simulink model "PubIfDecisionTOS_MDL"  (R2020b)
settings: configuration reference "DspaceConfig" (kept outside this file)
PostLoadFcn:
  | if any(exist('dsrtsu_mdlpostloadfcn', 'file') ~= 0), dsrtsu_mdlpostloadfcn('Execute', bdroot); end
InitFcn:
  | , if any(exist('dsmpb_private', 'file') ~= 0), dsmpb_private('dsmpb_mdlclblib', 'Init', bdroot); end,
undefined symbols (not defined in the file or in its folder): C_TOS_ACCEgoRAxletoFbumplength_m, C_TOS_ACCTargetFront_Flag, C_TOS_AEBJAPedObjDxThre_Val, C_TOS_AEBJAPedObjDyThre_Val, C_TOS_AEBJATargetSize_Val, C_TOS_AEBJAVehObjDxThre_Val, C_TOS_AEBJAVehObjDyThre_Val, C_TOS_AEBJuncPedTargetSize_Val, C_TOS_AEBLatObjDxThre_Val, C_TOS_AEBLatPedDyThre_Val, C_TOS_AEBLatTargetSize_Val, C_TOS_AEBLongTargetInEgoFront_Flag, C_TOS_axAbsGround_Parameter, C_TOS_CameraConfirmedFlag, C_TOS_CNsubjWidth, C_TOS_CurrentLaneCoreMinWidth_Val, C_TOS_CutInProb_Val_Zero, C_TOS_CutOutProb_Val_Zero, C_TOS_D2R_Val, C_TOS_DefaultValueObjectToCenterLine_dy, C_TOS_EgoCarWidth_Val, C_TOS_EgoDxRefPoint_m, C_TOS_EgoRAxletoFbumplength_m, C_TOS_HalfWidthVehicle_Con, C_TOS_HWA_CurrentLaneFlag, C_TOS_HWA_LeftLaneFlag, C_TOS_HWA_MovingDir_Vaild, C_TOS_HWA_MovState_Vaild, C_TOS_HWA_RightLaneFlag, C_TOS_LaneLineCourseErrorFront, C_TOS_LaneLineCourseErrorRear, C_TOS_MotorbikeDefaultWidth_m, C_TOS_NumberOfEffectiveTargets, C_TOS_Obj_Age_Val, C_TOS_Objdx_Constraint_Val, C_TOS_ObjectDefaultWidth_m, C_TOS_ObjInCurrentLane_Val, C_TOS_ObjInCurrentLaneValid, C_TOS_ObjInLeftLaneValid, C_TOS_ObjInRightLaneValid, C_TOS_ObjNotInCurrentLane_Val, C_TOS_ObjNotREElementType, C_TOS_ObjPredictDis_dy_ConstantVal_Zeros, C_TOS_ObjToCenterLine_ConstantVal_Zeros, C_TOS_OFMObjIDInvilad_Val, C_TOS_PIL_LatDisCons_Val_zero, C_TOS_PIL_ObjectCutInFlag_b, C_TOS_PIL_ObjectCutOutFlag_b, C_TOS_PIL_ObjLaneProb_al_Val, C_TOS_PP_ObjFusType_FC_Confirm_b, C_TOS_PP_ObjFusType_FC_FR_Confirm_b, C_TOS_PP_ObjFusType_FR_Confirm_b, C_TOS_RE_80BoolDefault_Val, C_TOS_RE_80Single181Default_Val, C_TOS_RE_80Single255Default_Val, C_TOS_RE_80Uint8Default_Val, C_TOS_RE_D2R, C_TOS_RE_D_180_Val, C_TOS_RE_InvalidObjectID_Val, C_TOS_RE_InvalidTargetChainDir_Val ... (+142)
libraries: simulink x1650, TOS_LIB x361, canfdmsglib x14
(part 69 of 69)

== stateflow chart PubIfDecisionTOS_MDL/TOS_20201112/TOS_2012080320/TOS/LC_LCKie_ELK/HWA_TargetInfor/TOS_HWA_TargetInfor ==
  (default) -> (junction 140) : {i = uint8(1);}
  (junction 140) -> (junction 145) [order 1] : [i <= P_TOS_LCTargetNum_Val]
  (junction 147) -> (junction 140) : {i=i+uint8(1);}
  (junction 140) -> (junction 143) [order 2]
  (junction 145) -> (junction 147) : {
      | TOS_LCTargetInfor.Object_Fus_Type(i) = uint8(0);
      | TOS_LCTargetInfor.Object_ID(i) = uint8(0);
      | TOS_LCTargetInfor.Object_Type(i) = uint8(0);
      | TOS_LCTargetInfor.Object_Length(i) = single(0);
      | TOS_LCTargetInfor.Object_Width(i) = single(0);
      | TOS_LCTargetInfor.Object_Hight(i) =single(0);
      | TOS_LCTargetInfor.Object_HeadingAngle(i) =single(0);
      | TOS_LCTargetInfor.Object_YawAngle(i) = single(0);
      | TOS_LCTargetInfor.Object_MovingState(i) = uint8(0);
      | TOS_LCTargetInfor.Object_Orientation(i) = uint8(0);
      | TOS_LCTargetInfor.Object_DX(i) = single(0);
      | TOS_LCTargetInfor.Object_DY(i) = single(0);
      | TOS_LCTargetInfor.Object_VX(i) = single(0);
      | TOS_LCTargetInfor.Object_VY(i) = single(0);
      | TOS_LCTargetInfor.Object_Std_AX(i) = single(0);
      | TOS_LCTargetInfor.Object_Std_AY(i) = single(0);
      | TOS_LCTargetInfor.Object_Std_DX(i) = single(0);
      | TOS_LCTargetInfor.Object_Std_DY(i) = single(0);
      | TOS_LCTargetInfor.Object_Std_VX(i) = single(0);
      | TOS_LCTargetInfor.Object_Std_VY(i) = single(0);
      | TOS_LCTargetInfor.Object_AX(i) = single(0);
      | TOS_LCTargetInfor.Object_AY(i) = single(0);
      | TOS_LCTargetInfor.Object_Std_Length(i) = single(0);
      | TOS_LCTargetInfor.Object_Std_Width(i) = single(0);
      | TOS_LCTargetInfor.Object_Std_HeadingAngle(i) = single(0);
      | TOS_LCTargetInfor.Object_Type_Prob(i) = single(0);
      | TOS_LCTargetInfor.Object_ExistProb(i) = single(0);
      | TOS_LCTargetInfor.Object_ObstacleProb(i) = single(0);
      | TOS_LCTargetInfor.Object_Age(i) = uint16(0);
      | TOS_LCTargetInfor.CurrentLane_Prob(i) = single(0);
      | TOS_LCTargetInfor.LeftLane_Prob(i) = single(0);
      | TOS_LCTargetInfor.RightLane_Prob(i) = single(0);
      | TOS_LCTargetInfor.ObjectIn_Lane(i) = uint8(0);
      | }
  (junction 143) -> (junction 56)
  (junction 56) -> (junction 121) : {i=uint8(1);
      | TargetIndex = uint8(0);}
  (junction 121) -> (junction 122) [order 1] : [i <= P_TOS_LCTargetNum_Val]
  (junction 124) -> (junction 121) : {i=i+uint8(1);}
  (junction 121) -> (junction 127) [order 2]
  (junction 122) -> (junction 158)
  (junction 158) -> (junction 160) [order 1] : [TOS_HWA_TargetIndexVector(i)~=uint8(0)]
  (junction 158) -> (junction 163) [order 2]
  (junction 160) -> (junction 162) : {TargetIndex=TOS_HWA_TargetIndexVector(i);
      | TOS_LCTargetInfor.Object_Fus_Type(i) = OFM_SignalVerification.Object_Fus_Type(TargetIndex);
      | TOS_LCTargetInfor.Object_ID(i) = OFM_SignalVerification.Object_ID(TargetIndex);
      | TOS_LCTargetInfor.Object_Type(i) = OFM_SignalVerification.Object_Type(TargetIndex);
      | TOS_LCTargetInfor.Object_Length(i) = OFM_SignalVerification.Object_Length(TargetIndex);
      | TOS_LCTargetInfor.Object_Width(i) = OFM_SignalVerification.Object_Width(TargetIndex);
      | TOS_LCTargetInfor.Object_Hight(i) = OFM_SignalVerification.Object_Hight(TargetIndex);
      | TOS_LCTargetInfor.Object_HeadingAngle(i) = OFM_SignalVerification.Object_HeadingAngle(TargetIndex);
      | TOS_LCTargetInfor.Object_YawAngle(i) = OFM_SignalVerification.Object_YawAngle(TargetIndex);
      | TOS_LCTargetInfor.Object_MovingState(i) = TOS_AddAttributes.PP_MovingStateSignalProcessing(TargetIndex);
      | TOS_LCTargetInfor.Object_Orientation(i) = TOS_AddAttributes.PP_ObjMovingDirSignalProcessing(TargetIndex);
      | TOS_LCTargetInfor.Object_DX(i) = OFM_SignalVerification.Object_DX(TargetIndex);
      | TOS_LCTargetInfor.Object_DY(i) = OFM_SignalVerification.Object_DY(TargetIndex);
      | TOS_LCTargetInfor.Object_VX(i) = OFM_SignalVerification.Object_VX(TargetIndex);
      | TOS_LCTargetInfor.Object_VY(i) = OFM_SignalVerification.Object_VY(TargetIndex);
      | TOS_LCTargetInfor.Object_Std_AX(i) = OFM_SignalVerification.Object_Std_AX(TargetIndex);
      | TOS_LCTargetInfor.Object_Std_AY(i) = OFM_SignalVerification.Object_Std_AY(TargetIndex);
      | TOS_LCTargetInfor.Object_Std_DX(i) = OFM_SignalVerification.Object_Std_DX(TargetIndex);
      | TOS_LCTargetInfor.Object_Std_DY(i) = OFM_SignalVerification.Object_Std_DY(TargetIndex);
      | TOS_LCTargetInfor.Object_Std_VX(i) = OFM_SignalVerification.Object_Std_VX(TargetIndex);
      | TOS_LCTargetInfor.Object_Std_VY(i) = OFM_SignalVerification.Object_Std_VY(TargetIndex);
      | TOS_LCTargetInfor.Object_AX(i) = OFM_SignalVerification.Object_AX(TargetIndex);
      | TOS_LCTargetInfor.Object_AY(i) = OFM_SignalVerification.Object_AY(TargetIndex);
      | TOS_LCTargetInfor.Object_Std_Length(i) = OFM_SignalVerification.Object_Std_Length(TargetIndex);
      | TOS_LCTargetInfor.Object_Std_Width(i) = OFM_SignalVerification.Object_Std_Width(TargetIndex);
      | TOS_LCTargetInfor.Object_Std_HeadingAngle(i) = OFM_SignalVerification.Object_Std_HeadingAngle(TargetIndex);
      | TOS_LCTargetInfor.Object_Type_Prob(i) = OFM_SignalVerification.Object_Type_Prob(TargetIndex);
      | TOS_LCTargetInfor.Object_ExistProb(i) = OFM_SignalVerification.Object_ExistProb(TargetIndex);
      | TOS_LCTargetInfor.Object_ObstacleProb(i) = OFM_SignalVerification.Object_ObstacleProb(TargetIndex);
      | TOS_LCTargetInfor.Object_Age(i) = OFM_SignalVerification.Object_Age(TargetIndex);
      | TOS_LCTargetInfor.CurrentLane_Prob(i) = TOS_ProbInLaneCalculat.PIL_CurrentLaneProb(TargetIndex);
      | TOS_LCTargetInfor.LeftLane_Prob(i) = TOS_ProbInLaneCalculat.PIL_LeftLaneProb(TargetIndex);
      | TOS_LCTargetInfor.RightLane_Prob(i) = TOS_ProbInLaneCalculat.PIL_RightLaneProb(TargetIndex);
      | TOS_LCTargetInfor.ObjectIn_Lane(i) =  ObjectIn_Lane_b(i);
      | }
  (junction 162) -> (junction 163)
  (junction 163) -> (junction 124)
  (junction 127) -> (junction 129)
  data: OFM_SignalVerification input Bus: OFM_OBJ_BUS; TOS_AddAttributes input Bus: TOS_AddAttributes_BUS; TOS_ProbInLaneCalculat input Bus: PIL_ProbInLaneCalculat_BUS; ObjectIn_Lane_b input uint8; TOS_HWA_TargetIndexVector input size=11; TOS_LCTargetInfor output Bus: TOS_LC_BUS size=1 =0; P_TOS_LCTargetNum_Val parameter uint8; TargetIndex local uint8 size=1; i local uint8 size=1

== stateflow chart PubIfDecisionTOS_MDL/TOS_20201112/TOS_2012080320/TOS/LC_LCKie_ELK/LCKie_TargetInfor/TOS_LCKieTargetInfor ==
  (default) -> (junction 161) : {i = uint8(1);}
  (junction 161) -> (junction 166) [order 1] : [i <= P_TOS_LCKieTargetNum_Val]
  (junction 169) -> (junction 161) : {i=i+uint8(1);}
  (junction 161) -> (junction 157) [order 2]
  (junction 166) -> (junction 169) : {
      | TOS_LCKieTargetInfor.Object_Fus_Type(i) = uint8(0);
      | TOS_LCKieTargetInfor.Object_ID(i) = uint8(0);
      | TOS_LCKieTargetInfor.Object_Type(i) = uint8(0);
      | TOS_LCKieTargetInfor.Object_Length(i) = single(0);
      | TOS_LCKieTargetInfor.Object_Width(i) = single(0);
      | TOS_LCKieTargetInfor.Object_Hight(i) =single(0);
      | TOS_LCKieTargetInfor.Object_HeadingAngle(i) =single(0);
      | TOS_LCKieTargetInfor.Object_YawAngle(i) = single(0);
      | TOS_LCKieTargetInfor.Object_MovingState(i) = uint8(0);
      | TOS_LCKieTargetInfor.Object_Orientation(i) = uint8(0);
      | TOS_LCKieTargetInfor.Object_DX(i) = single(0);
      | TOS_LCKieTargetInfor.Object_DY(i) = single(0);
      | TOS_LCKieTargetInfor.Object_VX(i) = single(0);
      | TOS_LCKieTargetInfor.Object_VY(i) = single(0);
      | TOS_LCKieTargetInfor.Object_Std_AX(i) = single(0);
      | TOS_LCKieTargetInfor.Object_Std_AY(i) = single(0);
      | TOS_LCKieTargetInfor.Object_Std_DX(i) = single(0);
      | TOS_LCKieTargetInfor.Object_Std_DY(i) = single(0);
      | TOS_LCKieTargetInfor.Object_Std_VX(i) = single(0);
      | TOS_LCKieTargetInfor.Object_Std_VY(i) = single(0);
      | TOS_LCKieTargetInfor.Object_AX(i) = single(0);
      | TOS_LCKieTargetInfor.Object_AY(i) = single(0);
      | TOS_LCKieTargetInfor.Object_Std_Length(i) = single(0);
      | TOS_LCKieTargetInfor.Object_Std_Width(i) = single(0);
      | TOS_LCKieTargetInfor.Object_Std_HeadingAngle(i) = single(0);
      | TOS_LCKieTargetInfor.Object_Type_Prob(i) = single(0);
      | TOS_LCKieTargetInfor.Object_ExistProb(i) = single(0);
      | TOS_LCKieTargetInfor.Object_ObstacleProb(i) = single(0);
      | TOS_LCKieTargetInfor.Object_Age(i) = uint16(0);
      | TOS_LCKieTargetInfor.cutIn(i) = uint8(0);
      | TOS_LCKieTargetInfor.CurrentLane_Prob(i) = single(0);
      | TOS_LCKieTargetInfor.LeftLane_Prob(i) = single(0);
      | TOS_LCKieTargetInfor.RightLane_Prob(i) = single(0);
      | TOS_LCKieTargetInfor.ObjectIn_Lane(i) = uint8(0);
      | }
  (junction 157) -> (junction 178)
  (junction 178) -> (junction 184) : {i=uint8(1);
      | TargetIndex = uint8(0);}
  (junction 184) -> (junction 155) [order 1] : [i <= P_TOS_LCKieTargetNum_Val]
  (junction 180) -> (junction 184) : {i=i+uint8(1);}
  (junction 184) -> (junction 181) [order 2]
  (junction 155) -> (junction 174)
  (junction 174) -> (junction 159) [order 1] : [TOS_HWA_TargetIndexVector(i)~=uint8(0)]
  (junction 174) -> (junction 170) [order 2]
  (junction 159) -> (junction 173) : {TargetIndex=TOS_HWA_TargetIndexVector(i);
      | TOS_LCKieTargetInfor.Object_Fus_Type(i) = OFM_SignalVerification.Object_Fus_Type(TargetIndex);
      | TOS_LCKieTargetInfor.Object_ID(i) = OFM_SignalVerification.Object_ID(TargetIndex);
      | TOS_LCKieTargetInfor.Object_Type(i) = OFM_SignalVerification.Object_Type(TargetIndex);
      | TOS_LCKieTargetInfor.Object_Length(i) = OFM_SignalVerification.Object_Length(TargetIndex);
      | TOS_LCKieTargetInfor.Object_Width(i) = OFM_SignalVerification.Object_Width(TargetIndex);
      | TOS_LCKieTargetInfor.Object_Hight(i) = OFM_SignalVerification.Object_Hight(TargetIndex);
      | TOS_LCKieTargetInfor.Object_HeadingAngle(i) = OFM_SignalVerification.Object_HeadingAngle(TargetIndex);
      | TOS_LCKieTargetInfor.Object_YawAngle(i) = OFM_SignalVerification.Object_YawAngle(TargetIndex);
      | TOS_LCKieTargetInfor.Object_MovingState(i) = TOS_AddAttributes.PP_MovingStateSignalProcessing(TargetIndex);
      | TOS_LCKieTargetInfor.Object_Orientation(i) = TOS_AddAttributes.PP_ObjMovingDirSignalProcessing(TargetIndex);
      | TOS_LCKieTargetInfor.Object_DX(i) = OFM_SignalVerification.Object_DX(TargetIndex);
      | TOS_LCKieTargetInfor.Object_DY(i) = OFM_SignalVerification.Object_DY(TargetIndex);
      | TOS_LCKieTargetInfor.Object_VX(i) = OFM_SignalVerification.Object_VX(TargetIndex);
      | TOS_LCKieTargetInfor.Object_VY(i) = OFM_SignalVerification.Object_VY(TargetIndex);
      | TOS_LCKieTargetInfor.Object_Std_AX(i) = OFM_SignalVerification.Object_Std_AX(TargetIndex);
      | TOS_LCKieTargetInfor.Object_Std_AY(i) = OFM_SignalVerification.Object_Std_AY(TargetIndex);
      | TOS_LCKieTargetInfor.Object_Std_DX(i) = OFM_SignalVerification.Object_Std_DX(TargetIndex);
      | TOS_LCKieTargetInfor.Object_Std_DY(i) = OFM_SignalVerification.Object_Std_DY(TargetIndex);
      | TOS_LCKieTargetInfor.Object_Std_VX(i) = OFM_SignalVerification.Object_Std_VX(TargetIndex);
      | TOS_LCKieTargetInfor.Object_Std_VY(i) = OFM_SignalVerification.Object_Std_VY(TargetIndex);
      | TOS_LCKieTargetInfor.Object_AX(i) = OFM_SignalVerification.Object_AX(TargetIndex);
      | TOS_LCKieTargetInfor.Object_AY(i) = OFM_SignalVerification.Object_AY(TargetIndex);
      | TOS_LCKieTargetInfor.Object_Std_Length(i) = OFM_SignalVerification.Object_Std_Length(TargetIndex);
      | TOS_LCKieTargetInfor.Object_Std_Width(i) = OFM_SignalVerification.Object_Std_Width(TargetIndex);
      | TOS_LCKieTargetInfor.Object_Std_HeadingAngle(i) = OFM_SignalVerification.Object_Std_HeadingAngle(TargetIndex);
      | TOS_LCKieTargetInfor.Object_Type_Prob(i) = OFM_SignalVerification.Object_Type_Prob(TargetIndex);
      | TOS_LCKieTargetInfor.Object_ExistProb(i) = OFM_SignalVerification.Object_ExistProb(TargetIndex);
      | TOS_LCKieTargetInfor.Object_ObstacleProb(i) = OFM_SignalVerification.Object_ObstacleProb(TargetIndex);
      | TOS_LCKieTargetInfor.Object_Age(i) = OFM_SignalVerification.Object_Age(TargetIndex);
      | TOS_LCKieTargetInfor.cutIn(i) =TOS_ProbInLaneCalculat.PIL_CutinFlag(TargetIndex) ;
      | TOS_LCKieTargetInfor.CurrentLane_Prob(i) = TOS_ProbInLaneCalculat.PIL_CurrentLaneProb(TargetIndex);
      | TOS_LCKieTargetInfor.LeftLane_Prob(i) = TOS_ProbInLaneCalculat.PIL_LeftLaneProb(TargetIndex);
      | TOS_LCKieTargetInfor.RightLane_Prob(i) = TOS_ProbInLaneCalculat.PIL_RightLaneProb(TargetIndex);
      | TOS_LCKieTargetInfor.ObjectIn_Lane(i) = ObjectIn_Lane_b(i);
      | }
  (junction 173) -> (junction 170)
  (junction 170) -> (junction 180)
  (junction 181) -> (junction 158)
  data: OFM_SignalVerification input Bus: OFM_OBJ_BUS; TOS_AddAttributes input Bus: TOS_AddAttributes_BUS; TOS_ProbInLaneCalculat input Bus: PIL_ProbInLaneCalculat_BUS; ObjectIn_Lane_b input uint8; TOS_HWA_TargetIndexVector input size=11; TOS_LCKieTargetInfor output Bus: TOS_LCKIE_BUS size=1 =0; P_TOS_LCKieTargetNum_Val parameter uint8; TargetIndex local uint8 size=1; i local uint8 size=1

== matlab function PubIfDecisionTOS_MDL/TOS_20201112/TOS_2012080320/TOS/LC_LCKie_ELK/TOS_HWA/CurrentLane/HWA_CurrentLane ==
  data: F_Dx2edNearestObjIndex output; Object_Dx input; Object_ID input; F_Dx1stNearestObjIndex output; R_Dx1stNearestObjIndex output; R_Dx2edNearestObjIndex output; F_Dx1stNearestObjID output; F_Dx2edNearestObjID output; ConditionJudge input; TOS_HWA_CLF_TargetPre_Filt_Flag input; Object_Num input; R_Dx1stNearestObjID output; R_Dx2edNearestObjID output

%%%%ObjDisIndex按Dx从小到大的总排序
%%%%%%%%ObjectID按Dx从小到大的总排序
function [F_Dx2edNearestObjIndex,F_Dx1stNearestObjIndex,R_Dx1stNearestObjIndex,R_Dx2edNearestObjIndex,F_Dx1stNearestObjID,F_Dx2edNearestObjID,R_Dx1stNearestObjID,R_Dx2edNearestObjID]   = MinMax(Object_Dx,Object_ID,ConditionJudge,TOS_HWA_CLF_TargetPre_Filt_Flag, Object_Num)
Dx_Front = Object_Dx;
Dx_Rear = Object_Dx;
ID = Object_ID;
for i=int32(1):int32(Object_Num)
    
    if (ID(i) == uint8(0))||(ConditionJudge(i) == false)||(Dx_Front(i) < single(0)) ||(TOS_HWA_CLF_TargetPre_Filt_Flag(i) == false)%%%%%本车道/前方/非0目标
       Dx_Front(i) = single(255);
    end
    
end

[F_MinDx1st,F_MinIndex1st] = min(Dx_Front);
if (F_MinDx1st > single(250))
   F_Dx1stNearestObjIndex = uint8(0);
   F_Dx1stNearestObjID = uint8(0); 
   F_Dx2edNearestObjIndex = uint8(0);
   F_Dx2edNearestObjID = uint8(0);
else
    Dx_Front(F_MinIndex1st) = single(255);
    [MinDx2ed,MinIndex2ed] = min(Dx_Front);
    F_Dx1stNearestObjIndex = uint8(F_MinIndex1st);
    F_Dx1stNearestObjID = uint8(ID(F_MinIndex1st)); 
   
   if (MinDx2ed > single(250))
     F_Dx2edNearestObjIndex = uint8(0);
     F_Dx2edNearestObjID = uint8(0);
   else
     F_Dx2edNearestObjIndex = uint8(MinIndex2ed);
     F_Dx2edNearestObjID = uint8(ID(MinIndex2ed));
   end
   

end

for i=int32(1):int32(Object_Num)
    
    if (ID(i) == uint8(0))||(ConditionJudge(i) == false)||(Dx_Rear(i) >= single(0))%%%%%本车道/后方/非0目标
       Dx_Rear(i) = single(255);
    end
    
end
Dx_Rear = abs(Dx_Rear);

[R_MinDx1st,R_MinIndex1st] = min(Dx_Rear);
if (R_MinDx1st > single(250))
   R_Dx1stNearestObjIndex = uint8(0);
   R_Dx1stNearestObjID = uint8(0); 
   R_Dx2edNearestObjIndex = uint8(0);
   R_Dx2edNearestObjID = uint8(0);
else
    Dx_Rear(R_MinIndex1st) = single(255);
    [R_MinDx2ed,R_MinIndex2ed] = min(Dx_Rear);
    R_Dx1stNearestObjIndex = uint8(R_MinIndex1st);
    R_Dx1stNearestObjID = uint8(ID(R_MinIndex1st)); 
   
   if (R_MinDx2ed > single(250))
     R_Dx2edNearestObjIndex = uint8(0);
     R_Dx2edNearestObjID = uint8(0);
   else
     R_Dx2edNearestObjIndex = uint8(R_MinIndex2ed);
     R_Dx2edNearestObjID = uint8(ID(R_MinIndex2ed));
   end

end

end

== stateflow chart PubIfDecisionTOS_MDL/TOS_20201112/TOS_2012080320/TOS/LC_LCKie_ELK/TOS_HWA/CurrentLane/HWA_CurrentLane_Target/HWA_CLF_Target_1/HWA_CLF_Target/HWA_CLF_Target/HWA_CLF_FusionTypeConfirm/Subsystem1/TOS_ObjMovStateCfmFlow1 ==
  note: TOS_ObjMovStateCfm Coding:
      | 0: Object default moving state
      | 1：Object had been moving
      | 2: Object is moving
  (default) -> (junction 1)
  (junction 1) -> (junction 3) [order 1] : [Target_ID_K1 ~=C_TOS_OFMObjIDInvilad_Val&&...
      | Target_ID_K2 ~= C_TOS_OFMObjIDInvilad_Val]
  (junction 1) -> (junction 38) [order 2] : {
      |   TOS_ObjMovStateCfm = uint8(0);
      | }
  (junction 3) -> (junction 5)
  (junction 5) -> (junction 7) [order 1] : [Target_ID_K1 ==Target_ID_K2]
  (junction 5) -> (junction 35) [order 2] : {
      |   TOS_ObjMovStateCfm =uint8(0);
      | }
  (junction 7) -> (junction 9)
  (junction 9) -> (junction 11) [order 1] : [ObjectID ==Target_ID_K1]
  (junction 9) -> (junction 29) [order 2] : {
      |   TOS_ObjMovStateCfm = uint8(0);
      | }
  (junction 11) -> (junction 13)
  (junction 13) -> (junction 15) [order 1] : [(Target_MovState_K2 == ObjectMovingState_E.Moving||...
      | Target_MovState_K2 == ObjectMovingState_E.Stopped)&&...
      | (Target_MovState_K1 == ObjectMovingState_E.Moving||...
      | Target_MovState_K1 == ObjectMovingState_E.Stopped)||...
      |   TOS_ObjMovStateCfm == uint8(1)]
  (junction 13) -> (junction 52) [order 2]
  (junction 15) -> (junction 58) : {
      |   TOS_ObjMovStateCfm = uint8(1);
      | }
  (junction 52) -> (junction 23) [order 1] : [ObjMovState == OFM_OBJ_MOVINGSTATE_E.STOPPED||...
      | ObjMovState == OFM_OBJ_MOVINGSTATE_E.MOVING]
  (junction 52) -> (junction 27) [order 2] : {
      |   TOS_ObjMovStateCfm = uint8(0);
      | }
  (junction 23) -> (junction 54) : {
      |   TOS_ObjMovStateCfm = uint8(2);
      | }
  (junction 35) -> (junction 38)
  (junction 29) -> (junction 35)
  (junction 27) -> (junction 29)
  (junction 54) -> (junction 27)
  (junction 58) -> (junction 54)
  (junction 38) -> (junction 41)
  data: Target_ID_K1 input uint8; Target_ID_K2 input uint8; Target_MovState_K1 input Enum: ObjectMovingState_E; Target_MovState_K2 input Enum: ObjectMovingState_E; ObjMovState input Enum: OFM_OBJ_MOVINGSTATE_E; ObjectID input uint8; TOS_ObjMovStateCfm output uint8; C_TOS_OFMObjIDInvilad_Val parameter uint8

== stateflow chart PubIfDecisionTOS_MDL/TOS_20201112/TOS_2012080320/TOS/LC_LCKie_ELK/TOS_HWA/CurrentLane/HWA_CurrentLane_Target/HWA_CLF_Target_1/HWA_CLF_Target/HWA_CLF_Target/HWA_CLF_ObjTypeConfirm/Subsystem/TOS_ObjMovStateCfmFlow1 ==
  note: TOS_ObjMovStateCfm Coding:
      | 0: Object default moving state
      | 1：Object had been moving
      | 2: Object is moving
  (default) -> (junction 1)
  (junction 1) -> (junction 3) [order 1] : [ACC_TargetP0_ID_K1 ~=C_TOS_OFMObjIDInvilad_Val&&...
      | ACC_TargetP0_ID_K2 ~= C_TOS_OFMObjIDInvilad_Val]
  (junction 1) -> (junction 38) [order 2] : {
      |   TOS_ObjMovStateCfm = uint8(0);
      | }
  (junction 3) -> (junction 5)
  (junction 5) -> (junction 7) [order 1] : [ACC_TargetP0_ID_K1 ==ACC_TargetP0_ID_K2]
  (junction 5) -> (junction 35) [order 2] : {
      |   TOS_ObjMovStateCfm =uint8(0);
      | }
  (junction 7) -> (junction 9)
  (junction 9) -> (junction 11) [order 1] : [ObjectID ==ACC_TargetP0_ID_K1]
  (junction 9) -> (junction 29) [order 2] : {
      |   TOS_ObjMovStateCfm = uint8(0);
      | }
  (junction 11) -> (junction 13)
  (junction 13) -> (junction 15) [order 1] : [(ACC_TargetP0_MovState_K2 == ObjectMovingState_E.Moving||...
      | ACC_TargetP0_MovState_K2 == ObjectMovingState_E.Stopped)&&...
      | (ACC_TargetP0_MovState_K1 == ObjectMovingState_E.Moving||...
      | ACC_TargetP0_MovState_K1 == ObjectMovingState_E.Stopped)||...
      |   TOS_ObjMovStateCfm == uint8(1)]
  (junction 13) -> (junction 52) [order 2]
  (junction 15) -> (junction 58) : {
      |   TOS_ObjMovStateCfm = uint8(1);
      | }
  (junction 52) -> (junction 23) [order 1] : [ObjMovState == OFM_OBJ_MOVINGSTATE_E.STOPPED||...
      | ObjMovState == OFM_OBJ_MOVINGSTATE_E.MOVING]
  (junction 52) -> (junction 27) [order 2] : {
      |   TOS_ObjMovStateCfm = uint8(0);
      | }
  (junction 23) -> (junction 54) : {
      |   TOS_ObjMovStateCfm = uint8(2);
      | }
  (junction 35) -> (junction 38)
  (junction 29) -> (junction 35)
  (junction 27) -> (junction 29)
  (junction 54) -> (junction 27)
  (junction 58) -> (junction 54)
  (junction 38) -> (junction 41)
  data: ACC_TargetP0_ID_K1 input uint8; ACC_TargetP0_ID_K2 input uint8; ACC_TargetP0_MovState_K1 input Enum: ObjectMovingState_E; ACC_TargetP0_MovState_K2 input Enum: ObjectMovingState_E; ObjMovState input Enum: OFM_OBJ_MOVINGSTATE_E; ObjectID input uint8; TOS_ObjMovStateCfm output uint8; C_TOS_OFMObjIDInvilad_Val parameter uint8

== stateflow chart PubIfDecisionTOS_MDL/TOS_20201112/TOS_2012080320/TOS/LC_LCKie_ELK/TOS_HWA/CurrentLane/HWA_CurrentLane_Target/HWA_CLF_Target_1/HWA_CLF_Target/HWA_CLF_Target/HWA_CLF_TargetMovingDirConfirm/Subsystem/TOS_ObjMovStateCfmFlow ==
  note: TOS_ObjMovStateCfm Coding:
      | 0: Object default moving state
      | 1：Object had been moving
      | 2: Object had been Stopped
  (default) -> (junction 1)
  (junction 1) -> (junction 3) [order 1] : [Target_ID_K1 ~=C_TOS_OFMObjIDInvilad_Val&&...
      | Target_ID_K2 ~= C_TOS_OFMObjIDInvilad_Val]
  (junction 1) -> (junction 38) [order 2] : {
      |   TOS_ObjMovStateCfm = uint8(0);
      | }
  (junction 3) -> (junction 5)
  (junction 5) -> (junction 7) [order 1] : [Target_ID_K1 ==Target_ID_K2]
  (junction 5) -> (junction 35) [order 2] : {
      |   TOS_ObjMovStateCfm =uint8(0);
      | }
  (junction 7) -> (junction 9)
  (junction 9) -> (junction 11) [order 1] : [ObjectID ==Target_ID_K1]
  (junction 9) -> (junction 29) [order 2] : {
      |   TOS_ObjMovStateCfm = uint8(0);
      | }
  (junction 11) -> (junction 13)
  (junction 13) -> (junction 15) [order 1] : [Target_MovState_K2 == ObjectMovingState_E.Moving&&...
      | Target_MovState_K1 == ObjectMovingState_E.Moving||...
      |   TOS_ObjMovStateCfm == uint8(1)]
  (junction 13) -> (junction 52) [order 2]
  (junction 15) -> (junction 58) : {
      |   TOS_ObjMovStateCfm = uint8(1);
      | }
  (junction 52) -> (junction 23) [order 1] : [Target_MovState_K2 == ObjectMovingState_E.Stopped&&...
      | Target_MovState_K1 == ObjectMovingState_E.Stopped||...
      |   TOS_ObjMovStateCfm == uint8(2)]
  (junction 52) -> (junction 27) [order 2] : {
      |   TOS_ObjMovStateCfm = uint8(0);
      | }
  (junction 23) -> (junction 54) : {
      |   TOS_ObjMovStateCfm = uint8(2);
      | }
  (junction 35) -> (junction 38)
  (junction 29) -> (junction 35)
  (junction 27) -> (junction 29)
  (junction 54) -> (junction 27)
  (junction 58) -> (junction 54)
  (junction 38) -> (junction 41)
  data: Target_ID_K1 input uint8; Target_ID_K2 input uint8; Target_MovState_K1 input Enum: ObjectMovingState_E; Target_MovState_K2 input Enum: ObjectMovingState_E; ObjMovState input Enum: OFM_OBJ_MOVINGSTATE_E; ObjectID input uint8; TOS_ObjMovStateCfm output uint8; C_TOS_OFMObjIDInvilad_Val parameter uint8

== stateflow chart PubIfDecisionTOS_MDL/TOS_20201112/TOS_2012080320/TOS/LC_LCKie_ELK/TOS_HWA/CurrentLane/HWA_CurrentLane_Target/HWA_CLF_Target_2/HWA_CLF_Target/HWA_CLF_Target/HWA_CLF_FusionTypeConfirm/Subsystem1/TOS_ObjMovStateCfmFlow1 ==
  note: TOS_ObjMovStateCfm Coding:
      | 0: Object default moving state
      | 1：Object had been moving
      | 2: Object is moving
  (default) -> (junction 1)
  (junction 1) -> (junction 3) [order 1] : [Target_ID_K1 ~=C_TOS_OFMObjIDInvilad_Val&&...
      | Target_ID_K2 ~= C_TOS_OFMObjIDInvilad_Val]
  (junction 1) -> (junction 38) [order 2] : {
      |   TOS_ObjMovStateCfm = uint8(0);
      | }
  (junction 3) -> (junction 5)
  (junction 5) -> (junction 7) [order 1] : [Target_ID_K1 ==Target_ID_K2]
  (junction 5) -> (junction 35) [order 2] : {
      |   TOS_ObjMovStateCfm =uint8(0);
      | }
  (junction 7) -> (junction 9)
  (junction 9) -> (junction 11) [order 1] : [ObjectID ==Target_ID_K1]
  (junction 9) -> (junction 29) [order 2] : {
      |   TOS_ObjMovStateCfm = uint8(0);
      | }
  (junction 11) -> (junction 13)
  (junction 13) -> (junction 15) [order 1] : [(Target_MovState_K2 == ObjectMovingState_E.Moving||...
      | Target_MovState_K2 == ObjectMovingState_E.Stopped)&&...
      | (Target_MovState_K1 == ObjectMovingState_E.Moving||...
      | Target_MovState_K1 == ObjectMovingState_E.Stopped)||...
      |   TOS_ObjMovStateCfm == uint8(1)]
  (junction 13) -> (junction 52) [order 2]
  (junction 15) -> (junction 58) : {
      |   TOS_ObjMovStateCfm = uint8(1);
      | }
  (junction 52) -> (junction 23) [order 1] : [ObjMovState == OFM_OBJ_MOVINGSTATE_E.STOPPED||...
      | ObjMovState == OFM_OBJ_MOVINGSTATE_E.MOVING]
  (junction 52) -> (junction 27) [order 2] : {
      |   TOS_ObjMovStateCfm = uint8(0);
      | }
  (junction 23) -> (junction 54) : {
      |   TOS_ObjMovStateCfm = uint8(2);
      | }
  (junction 35) -> (junction 38)
  (junction 29) -> (junction 35)
  (junction 27) -> (junction 29)
  (junction 54) -> (junction 27)
  (junction 58) -> (junction 54)
  (junction 38) -> (junction 41)
  data: Target_ID_K1 input uint8; Target_ID_K2 input uint8; Target_MovState_K1 input Enum: ObjectMovingState_E; Target_MovState_K2 input Enum: ObjectMovingState_E; ObjMovState input Enum: OFM_OBJ_MOVINGSTATE_E; ObjectID input uint8; TOS_ObjMovStateCfm output uint8; C_TOS_OFMObjIDInvilad_Val parameter uint8

== stateflow chart PubIfDecisionTOS_MDL/TOS_20201112/TOS_2012080320/TOS/LC_LCKie_ELK/TOS_HWA/CurrentLane/HWA_CurrentLane_Target/HWA_CLF_Target_2/HWA_CLF_Target/HWA_CLF_Target/HWA_CLF_ObjTypeConfirm/Subsystem/TOS_ObjMovStateCfmFlow1 ==
  note: TOS_ObjMovStateCfm Coding:
      | 0: Object default moving state
      | 1：Object had been moving
      | 2: Object is moving
  (default) -> (junction 1)
  (junction 1) -> (junction 3) [order 1] : [ACC_TargetP0_ID_K1 ~=C_TOS_OFMObjIDInvilad_Val&&...
      | ACC_TargetP0_ID_K2 ~= C_TOS_OFMObjIDInvilad_Val]
  (junction 1) -> (junction 38) [order 2] : {
      |   TOS_ObjMovStateCfm = uint8(0);
      | }
  (junction 3) -> (junction 5)
  (junction 5) -> (junction 7) [order 1] : [ACC_TargetP0_ID_K1 ==ACC_TargetP0_ID_K2]
  (junction 5) -> (junction 35) [order 2] : {
      |   TOS_ObjMovStateCfm =uint8(0);
      | }
  (junction 7) -> (junction 9)
  (junction 9) -> (junction 11) [order 1] : [ObjectID ==ACC_TargetP0_ID_K1]
  (junction 9) -> (junction 29) [order 2] : {
      |   TOS_ObjMovStateCfm = uint8(0);
      | }
  (junction 11) -> (junction 13)
  (junction 13) -> (junction 15) [order 1] : [(ACC_TargetP0_MovState_K2 == ObjectMovingState_E.Moving||...
      | ACC_TargetP0_MovState_K2 == ObjectMovingState_E.Stopped)&&...
      | (ACC_TargetP0_MovState_K1 == ObjectMovingState_E.Moving||...
      | ACC_TargetP0_MovState_K1 == ObjectMovingState_E.Stopped)||...
      |   TOS_ObjMovStateCfm == uint8(1)]
  (junction 13) -> (junction 52) [order 2]
  (junction 15) -> (junction 58) : {
      |   TOS_ObjMovStateCfm = uint8(1);
      | }
  (junction 52) -> (junction 23) [order 1] : [ObjMovState == OFM_OBJ_MOVINGSTATE_E.STOPPED||...
      | ObjMovState == OFM_OBJ_MOVINGSTATE_E.MOVING]
  (junction 52) -> (junction 27) [order 2] : {
      |   TOS_ObjMovStateCfm = uint8(0);
      | }
  (junction 23) -> (junction 54) : {
      |   TOS_ObjMovStateCfm = uint8(2);
      | }
  (junction 35) -> (junction 38)
  (junction 29) -> (junction 35)
  (junction 27) -> (junction 29)
  (junction 54) -> (junction 27)
  (junction 58) -> (junction 54)
  (junction 38) -> (junction 41)
  data: ACC_TargetP0_ID_K1 input uint8; ACC_TargetP0_ID_K2 input uint8; ACC_TargetP0_MovState_K1 input Enum: ObjectMovingState_E; ACC_TargetP0_MovState_K2 input Enum: ObjectMovingState_E; ObjMovState input Enum: OFM_OBJ_MOVINGSTATE_E; ObjectID input uint8; TOS_ObjMovStateCfm output uint8; C_TOS_OFMObjIDInvilad_Val parameter uint8

== stateflow chart PubIfDecisionTOS_MDL/TOS_20201112/TOS_2012080320/TOS/LC_LCKie_ELK/TOS_HWA/CurrentLane/HWA_CurrentLane_Target/HWA_CLF_Target_2/HWA_CLF_Target/HWA_CLF_Target/HWA_CLF_TargetMovingDirConfirm/Subsystem/TOS_ObjMovStateCfmFlow ==
  note: TOS_ObjMovStateCfm Coding:
      | 0: Object default moving state
      | 1：Object had been moving
      | 2: Object had been Stopped
  (default) -> (junction 1)
  (junction 1) -> (junction 3) [order 1] : [Target_ID_K1 ~=C_TOS_OFMObjIDInvilad_Val&&...
      | Target_ID_K2 ~= C_TOS_OFMObjIDInvilad_Val]
  (junction 1) -> (junction 38) [order 2] : {
      |   TOS_ObjMovStateCfm = uint8(0);
      | }
  (junction 3) -> (junction 5)
  (junction 5) -> (junction 7) [order 1] : [Target_ID_K1 ==Target_ID_K2]
  (junction 5) -> (junction 35) [order 2] : {
      |   TOS_ObjMovStateCfm =uint8(0);
      | }
  (junction 7) -> (junction 9)
  (junction 9) -> (junction 11) [order 1] : [ObjectID ==Target_ID_K1]
  (junction 9) -> (junction 29) [order 2] : {
      |   TOS_ObjMovStateCfm = uint8(0);
      | }
  (junction 11) -> (junction 13)
  (junction 13) -> (junction 15) [order 1] : [Target_MovState_K2 == ObjectMovingState_E.Moving&&...
      | Target_MovState_K1 == ObjectMovingState_E.Moving||...
      |   TOS_ObjMovStateCfm == uint8(1)]
  (junction 13) -> (junction 52) [order 2]
  (junction 15) -> (junction 58) : {
      |   TOS_ObjMovStateCfm = uint8(1);
      | }
  (junction 52) -> (junction 23) [order 1] : [Target_MovState_K2 == ObjectMovingState_E.Stopped&&...
      | Target_MovState_K1 == ObjectMovingState_E.Stopped||...
      |   TOS_ObjMovStateCfm == uint8(2)]
  (junction 52) -> (junction 27) [order 2] : {
      |   TOS_ObjMovStateCfm = uint8(0);
      | }
  (junction 23) -> (junction 54) : {
      |   TOS_ObjMovStateCfm = uint8(2);
      | }
  (junction 35) -> (junction 38)
  (junction 29) -> (junction 35)
  (junction 27) -> (junction 29)
  (junction 54) -> (junction 27)
  (junction 58) -> (junction 54)
  (junction 38) -> (junction 41)
  data: Target_ID_K1 input uint8; Target_ID_K2 input uint8; Target_MovState_K1 input Enum: ObjectMovingState_E; Target_MovState_K2 input Enum: ObjectMovingState_E; ObjMovState input Enum: OFM_OBJ_MOVINGSTATE_E; ObjectID input uint8; TOS_ObjMovStateCfm output uint8; C_TOS_OFMObjIDInvilad_Val parameter uint8

== stateflow chart PubIfDecisionTOS_MDL/TOS_20201112/TOS_2012080320/TOS/LC_LCKie_ELK/TOS_HWA/CurrentLane/HWA_Object_PreConfirm/TOS_HWA_CurrentLaneFront_TargPreConfirm/TOS_HWA_CurrentLaneFront_TargPreConfirm/Subsystem3/Chart ==
  (default) -> (junction 1)
  (junction 1) -> (junction 3) [order 1] : [(FR_Confirm == C_TOS_PP_ObjFusType_FR_Confirm_b)&&...
      | ((Obj_MovingState == OFM_OBJ_MOVINGSTATE_E.STATIONARY)||...
      | (Obj_MovingState == OFM_OBJ_MOVINGSTATE_E.INVALID)||...
      | (Obj_MovingState == OFM_OBJ_MOVINGSTATE_E.UNKNOWN))]
  (junction 1) -> (junction 20) [order 2] : {
      |   ObjectisFence_Flag =false;
      | }
  (junction 3) -> (junction 5)
  (junction 5) -> (junction 35) [order 1] : [Object_ObstacleProb < single(0.85)]
  (junction 5) -> (junction 17) [order 2] : {
      |   ObjectisFence_Flag =false;
      | }
  (junction 35) -> (junction 37)
  (junction 37) -> (junction 39) [order 1] : [abs(Object_DY) < single(1.45) ]
  (junction 37) -> (junction 41) [order 2] : {
      |   ObjectisFence_Flag = true;
      | }
  (junction 39) -> (junction 15) : {
      |   ObjectisFence_Flag = false;
      | }
  (junction 17) -> (junction 20)
  (junction 41) -> (junction 17)
  (junction 15) -> (junction 41)
  (junction 20) -> (junction 23)
  data: FR_Confirm input boolean; Obj_MovingState input Enum: OFM_OBJ_MOVINGSTATE_E; ObjectisFence_Flag output boolean; Object_ObstacleProb input single; Object_DY input single; C_TOS_PP_ObjFusType_FR_Confirm_b parameter

== matlab function PubIfDecisionTOS_MDL/TOS_20201112/TOS_2012080320/TOS/LC_LCKie_ELK/TOS_HWA/LeftLane/HWA_LeftLane ==
  data: F_Dx2edNearestObjIndex output; Object_Dx input; Object_ID input; F_Dx1stNearestObjIndex output; R_Dx1stNearestObjIndex output; R_Dx2edNearestObjIndex output; F_Dx1stNearestObjID output; F_Dx2edNearestObjID output; ConditionJudge input; TOS_HWA_TargetPreConfirm input; Object_Num input; R_Dx1stNearestObjID output; R_Dx2edNearestObjID output
 
%%%%ObjDisIndex按Dx从小到大的总排序
%%%%%%%%ObjectID按Dx从小到大的总排序
function [F_Dx2edNearestObjIndex,F_Dx1stNearestObjIndex,R_Dx1stNearestObjIndex,R_Dx2edNearestObjIndex,F_Dx1stNearestObjID,F_Dx2edNearestObjID,R_Dx1stNearestObjID,R_Dx2edNearestObjID]   = MinMax(Object_Dx,Object_ID,ConditionJudge,TOS_HWA_TargetPreConfirm, Object_Num)
Dx_Front = Object_Dx;
Dx_Rear = Object_Dx;
ID = Object_ID;
for i=int32(1):int32(Object_Num)
    
    if (ID(i) == uint8(0))||(ConditionJudge(i) == false)||(Dx_Front(i) < single(0)) % ||(TOS_HWA_TargetPreConfirm(i) == false)%%%%%本车道/前方/非0目标
       Dx_Front(i) = single(255);
    end
    
end

[F_MinDx1st,F_MinIndex1st] = min(Dx_Front);
if (F_MinDx1st > single(250))
   F_Dx1stNearestObjIndex = uint8(0);
   F_Dx1stNearestObjID = uint8(0); 
   F_Dx2edNearestObjIndex = uint8(0);
   F_Dx2edNearestObjID = uint8(0);
else
    Dx_Front(F_MinIndex1st) = single(255);
    [MinDx2ed,MinIndex2ed] = min(Dx_Front);
    F_Dx1stNearestObjIndex = uint8(F_MinIndex1st);
    F_Dx1stNearestObjID = uint8(ID(F_MinIndex1st)); 
   
   if (MinDx2ed > single(250))
     F_Dx2edNearestObjIndex = uint8(0);
     F_Dx2edNearestObjID = uint8(0);
   else
     F_Dx2edNearestObjIndex = uint8(MinIndex2ed);
     F_Dx2edNearestObjID = uint8(ID(MinIndex2ed));
   end
   

end

for i=int32(1):int32(Object_Num)
    
    if (ID(i) == uint8(0))||(ConditionJudge(i) == false)||(Dx_Rear(i) >= single(0))%%%%%本车道/后方/非0目标
       Dx_Rear(i) = single(255);
    end
    
end
Dx_Rear = abs(Dx_Rear);

[R_MinDx1st,R_MinIndex1st] = min(Dx_Rear);
if (R_MinDx1st > single(250))
   R_Dx1stNearestObjIndex = uint8(0);
   R_Dx1stNearestObjID = uint8(0); 
   R_Dx2edNearestObjIndex = uint8(0);
   R_Dx2edNearestObjID = uint8(0);
else
    Dx_Rear(R_MinIndex1st) = single(255);
    [R_MinDx2ed,R_MinIndex2ed] = min(Dx_Rear);
    R_Dx1stNearestObjIndex = uint8(R_MinIndex1st);
    R_Dx1stNearestObjID = uint8(ID(R_MinIndex1st)); 
   
   if (R_MinDx2ed > single(250))
     R_Dx2edNearestObjIndex = uint8(0);
     R_Dx2edNearestObjID = uint8(0);
   else
     R_Dx2edNearestObjIndex = uint8(R_MinIndex2ed);
     R_Dx2edNearestObjID = uint8(ID(R_MinIndex2ed));
   end

end

end

== matlab function PubIfDecisionTOS_MDL/TOS_20201112/TOS_2012080320/TOS/LC_LCKie_ELK/TOS_HWA/RightLane/HWA_RightLane ==
  data: F_Dx2edNearestObjIndex output; Object_Dx input; Object_ID input; F_Dx1stNearestObjIndex output; R_Dx1stNearestObjIndex output; R_Dx2edNearestObjIndex output; F_Dx1stNearestObjID output; F_Dx2edNearestObjID output; ConditionJudge input; TOS_HWA_RLF_TargetPre_Confirm_Filt_Flag input; Object_Num input; R_Dx1stNearestObjID output; R_Dx2edNearestObjID output

%%%%ObjDisIndex按Dx从小到大的总排序
%%%%%%%%ObjectID按Dx从小到大的总排序
function [F_Dx2edNearestObjIndex,F_Dx1stNearestObjIndex,R_Dx1stNearestObjIndex,R_Dx2edNearestObjIndex,F_Dx1stNearestObjID,F_Dx2edNearestObjID,R_Dx1stNearestObjID,R_Dx2edNearestObjID]   = MinMax(Object_Dx,Object_ID,ConditionJudge,TOS_HWA_RLF_TargetPre_Confirm_Filt_Flag, Object_Num)
Dx_Front = Object_Dx;
Dx_Rear = Object_Dx;
ID = Object_ID;
for i=int32(1):int32(Object_Num)
    
    if (ID(i) == uint8(0))||(ConditionJudge(i) == false)||(Dx_Front(i) < single(0)) ||(TOS_HWA_RLF_TargetPre_Confirm_Filt_Flag(i) == false) %%%%%本车道/前方/非0目标
       Dx_Front(i) = single(255);
    end
    
end

[F_MinDx1st,F_MinIndex1st] = min(Dx_Front);
if (F_MinDx1st > single(250))
   F_Dx1stNearestObjIndex = uint8(0);
   F_Dx1stNearestObjID = uint8(0); 
   F_Dx2edNearestObjIndex = uint8(0);
   F_Dx2edNearestObjID = uint8(0);
else
    Dx_Front(F_MinIndex1st) = single(255);
    [MinDx2ed,MinIndex2ed] = min(Dx_Front);
    F_Dx1stNearestObjIndex = uint8(F_MinIndex1st);
    F_Dx1stNearestObjID = uint8(ID(F_MinIndex1st)); 
   
   if (MinDx2ed > single(250))
     F_Dx2edNearestObjIndex = uint8(0);
     F_Dx2edNearestObjID = uint8(0);
   else
     F_Dx2edNearestObjIndex = uint8(MinIndex2ed);
     F_Dx2edNearestObjID = uint8(ID(MinIndex2ed));
   end
   

end

for i=int32(1):int32(Object_Num)
    
    if (ID(i) == uint8(0))||(ConditionJudge(i) == false)||(Dx_Rear(i) >= single(0))%%%%%本车道/后方/非0目标
       Dx_Rear(i) = single(255);
    end
    
end
Dx_Rear = abs(Dx_Rear);

[R_MinDx1st,R_MinIndex1st] = min(Dx_Rear);
if (R_MinDx1st > single(250))
   R_Dx1stNearestObjIndex = uint8(0);
   R_Dx1stNearestObjID = uint8(0); 
   R_Dx2edNearestObjIndex = uint8(0);
   R_Dx2edNearestObjID = uint8(0);
else
    Dx_Rear(R_MinIndex1st) = single(255);
    [R_MinDx2ed,R_MinIndex2ed] = min(Dx_Rear);
    R_Dx1stNearestObjIndex = uint8(R_MinIndex1st);
    R_Dx1stNearestObjID = uint8(ID(R_MinIndex1st)); 
   
   if (R_MinDx2ed > single(250))
     R_Dx2edNearestObjIndex = uint8(0);
     R_Dx2edNearestObjID = uint8(0);
   else
     R_Dx2edNearestObjIndex = uint8(R_MinIndex2ed);
     R_Dx2edNearestObjID = uint8(ID(R_MinIndex2ed));
   end

end

end

== matlab function PubIfDecisionTOS_MDL/TOS_20201112/TOS_2012080320/TOS/P0_Trajectory_V1.0/DataConfirm/polyfit1 ==
  data: P0_dx_TrackRecord input; P0_dy_TrackRecord input; P0_StartPosition_Num input; P0_EndPosition_Num input; P0_Counter_TrackRecord input; P0_StartPosition_Dis input; P0_EndPosition_dx input; P0_EndPosition_dy input; P0_TrgValidConfirm_Counter input; VxvRef_ms input; OTL_Valid output size=1; OTL_C3 output size=1; OTL_C2 output; OTL_C1 output size=1; OTL_C0 output size=1; OTL_Range output size=1; OTL_Cnt output size=1; d_Start output; d_End output; P0_Counter output size=80; dy output size=80; P0_Trajectory_TrackRecord_Num input size=1; dx output size=80
function [ OTL_Valid,OTL_C3,OTL_C2,OTL_C1,OTL_C0,OTL_Range,OTL_Cnt,d_Start,d_End,P0_Counter,dy,dx] = ...
          fcn(P0_dx_TrackRecord,P0_dy_TrackRecord,P0_StartPosition_Num,P0_EndPosition_Num,P0_Counter_TrackRecord ,...
          P0_StartPosition_Dis, P0_EndPosition_dx, P0_EndPosition_dy, P0_TrgValidConfirm_Counter, VxvRef_ms, P0_Trajectory_TrackRecord_Num)

%%-----初始化-----     


P0_Trajectory_TrackRecord_Num = uint32(80);

dx=single(zeros(uint32(P0_Trajectory_TrackRecord_Num),1));
dy=single(zeros(uint32(P0_Trajectory_TrackRecord_Num),1));
P0_Counter=uint32(zeros(uint32(P0_Trajectory_TrackRecord_Num),1));

%%-----判断拟合点-----
if  P0_StartPosition_Num < P0_EndPosition_Num
    
  dx(uint32(1):(P0_Trajectory_TrackRecord_Num - P0_StartPosition_Num + uint32(1)),1)= P0_dx_TrackRecord(P0_StartPosition_Num:P0_Trajectory_TrackRecord_Num,1); 
  dy(uint32(1):(P0_Trajectory_TrackRecord_Num - P0_StartPosition_Num + uint32(1)),1)= P0_dy_TrackRecord(P0_StartPosition_Num:P0_Trajectory_TrackRecord_Num,1);
  P0_Counter(uint32(1):(P0_Trajectory_TrackRecord_Num - P0_StartPosition_Num + uint32(1)),1)= P0_Counter_TrackRecord(P0_StartPosition_Num:P0_Trajectory_TrackRecord_Num,1);
   
elseif P0_StartPosition_Num > P0_EndPosition_Num
    %前半段
  dx(uint32(1):(P0_Trajectory_TrackRecord_Num - P0_StartPosition_Num + uint32(1)),1)= P0_dx_TrackRecord(P0_StartPosition_Num:P0_Trajectory_TrackRecord_Num,1); 
  dy(uint32(1):(P0_Trajectory_TrackRecord_Num - P0_StartPosition_Num + uint32(1)),1)= P0_dy_TrackRecord(P0_StartPosition_Num:P0_Trajectory_TrackRecord_Num,1);  
  P0_Counter(uint32(1):(P0_Trajectory_TrackRecord_Num - P0_StartPosition_Num + uint32(1)),1)= P0_Counter_TrackRecord(P0_StartPosition_Num:P0_Trajectory_TrackRecord_Num,1);  
  
  %后半段
  dx((P0_Trajectory_TrackRecord_Num - P0_StartPosition_Num + uint32(2)):P0_Trajectory_TrackRecord_Num,1)= P0_dx_TrackRecord(uint32(1):(P0_StartPosition_Num-uint32(1)),1); 
  dy((P0_Trajectory_TrackRecord_Num - P0_StartPosition_Num + uint32(2)):P0_Trajectory_TrackRecord_Num,1)= P0_dy_TrackRecord(uint32(1):(P0_StartPosition_Num-uint32(1)),1);   
  P0_Counter((P0_Trajectory_TrackRecord_Num - P0_StartPosition_Num + uint32(2)):P0_Trajectory_TrackRecord_Num,1)= P0_Counter_TrackRecord(uint32(1):(P0_StartPosition_Num-uint32(1)),1);     
end

%-----无效目标位补齐------
for i= uint32(1) : P0_Trajectory_TrackRecord_Num
    
        if dx(i)==single(0) && dy(i)==single(0) && P0_Counter(i)==uint32(0) 
            dx(i)=P0_EndPosition_dx;
            dy(i)=P0_EndPosition_dy;
        end
   
end


%----------判断起始、终止位置----------------------
% [min_dx,index_dx_min] = min(dx);
[min_dx,~] = min(dx);
[max_dy,~] = max(dx);
 d_End = max_dy;
 d_Start = min_dx;

% d_End = P0_EndPosition_dx;
% d_Start = P0_StartPosition_Dis;

%-----P0存在生命周期----
OTL_Cnt=uint8(P0_TrgValidConfirm_Counter);


%-------dop range--------
OTL_Range = max_dy ;


%----------轨迹拟合----------------------
if d_Start< single(50) &&  VxvRef_ms >= 0.4166  && P0_TrgValidConfirm_Counter > uint8(5)
    P0_Trajectory_Line = polyfit(dx,dy,3);
    OTL_C3 = P0_Trajectory_Line(1);
    OTL_C2 = P0_Trajectory_Line(2);
    OTL_C1 = P0_Trajectory_Line(3);
    OTL_C0 = P0_Trajectory_Line(4); 
    OTL_Valid = true;
else
    OTL_C3=single(0);
    OTL_C2=single(0);
    OTL_C1=single(0);
    OTL_C0=single(0); 
    OTL_Valid = false;
end

== matlab function PubIfDecisionTOS_MDL/TOS_20201112/TOS_2012080320/TOS/P0_Trajectory_V1.0/TrackRecord/Subsystem1/MATLAB Function ==
  data: P0_dx_TrackRecord_CordinatConvert_K1 input; P0_dy_TrackRecord_CordinatConvert_K1 input; P0_Counter_TrackRecord_CordinatConvert_K1 input; P0_Trajectory_TrackRecord_Num input; EmptyDataConfirm output
function EmptyDataConfirm = fcn(P0_dx_TrackRecord_CordinatConvert_K1,P0_dy_TrackRecord_CordinatConvert_K1,P0_Counter_TrackRecord_CordinatConvert_K1,P0_Trajectory_TrackRecord_Num)

EmptyDataConfirm=false;

for i= uint32(1):P0_Trajectory_TrackRecord_Num
    
    if P0_dx_TrackRecord_CordinatConvert_K1(i)==single(0) && P0_dy_TrackRecord_CordinatConvert_K1(i)==single(0) && P0_Counter_TrackRecord_CordinatConvert_K1(i)==uint32(0)      
        EmptyDataConfirm=true;
        break;     
    end
    
    
end

== matlab function PubIfDecisionTOS_MDL/TOS_20201112/TOS_2012080320/TOS/P0_Trajectory_V1.0/TrackRecord/Subsystem1/MATLAB Function1 ==
  data: P0_dx_TrackRecord_CordinatConvert_K1 input; P0_dy_TrackRecord_CordinatConvert_K1 input; P0_Counter_TrackRecord_CordinatConvert_K1 input; P0_StartPosition_Num output; P0_StartPosition_Dis output; P0_EndPosition_Num output; P0_EndPosition_dx output; P0_EndPosition_dy output
function [P0_StartPosition_Num,P0_StartPosition_Dis,P0_EndPosition_Num,P0_EndPosition_dx,P0_EndPosition_dy] = fcn(P0_dx_TrackRecord_CordinatConvert_K1,P0_dy_TrackRecord_CordinatConvert_K1,P0_Counter_TrackRecord_CordinatConvert_K1)

%------
[~,index_Counter_min] = min(P0_Counter_TrackRecord_CordinatConvert_K1);  %起始位置
[~,index_Counter_max] = max(P0_Counter_TrackRecord_CordinatConvert_K1);  %终止位置

% -----起始位置
P0_StartPosition_Num = index_Counter_min;
P0_StartPosition_Dis = P0_dx_TrackRecord_CordinatConvert_K1(index_Counter_min);

% -----终止位置
P0_EndPosition_Num = index_Counter_max;
P0_EndPosition_dx = P0_dx_TrackRecord_CordinatConvert_K1(index_Counter_max);
P0_EndPosition_dy = P0_dy_TrackRecord_CordinatConvert_K1(index_Counter_max);

== matlab function PubIfDecisionTOS_MDL/TOS_20201112/TOS_2012080320/TOS/P0_Trajectory_V1.0/TrackRecord/Subsystem2/MATLAB Function ==
  data: P0_dx_TrackRecord_CordinatConvert_K1 input; P0_dy_TrackRecord_CordinatConvert_K1 input; P0_Counter_TrackRecord_CordinatConvert_K1 input; P0_Trajectory_TrackRecord_Num input; EmptyDataConfirm output
function EmptyDataConfirm = fcn(P0_dx_TrackRecord_CordinatConvert_K1,P0_dy_TrackRecord_CordinatConvert_K1,P0_Counter_TrackRecord_CordinatConvert_K1,P0_Trajectory_TrackRecord_Num)

EmptyDataConfirm=false;

for i= uint32(1):P0_Trajectory_TrackRecord_Num
    
    if P0_dx_TrackRecord_CordinatConvert_K1(i)==single(0) && P0_dy_TrackRecord_CordinatConvert_K1(i)==single(0) && P0_Counter_TrackRecord_CordinatConvert_K1(i)==uint32(0)      
        EmptyDataConfirm=true;
        break;     
    end
    
    
end

== matlab function PubIfDecisionTOS_MDL/TOS_20201112/TOS_2012080320/TOS/P0_Trajectory_V1.0/TrackRecord/Subsystem3/MATLAB Function ==
  data: P0_dx_TrackRecord_CordinatConvert_K1 input; P0_dy_TrackRecord_CordinatConvert_K1 input; P0_Counter_TrackRecord_CordinatConvert_K1 input; P0_Trajectory_TrackRecord_Num input; EmptyDataConfirm output
function EmptyDataConfirm = fcn(P0_dx_TrackRecord_CordinatConvert_K1,P0_dy_TrackRecord_CordinatConvert_K1,P0_Counter_TrackRecord_CordinatConvert_K1,P0_Trajectory_TrackRecord_Num)

EmptyDataConfirm=false;

for i= uint32(1):P0_Trajectory_TrackRecord_Num
    
    if P0_dx_TrackRecord_CordinatConvert_K1(i)==single(0) && P0_dy_TrackRecord_CordinatConvert_K1(i)==single(0) && P0_Counter_TrackRecord_CordinatConvert_K1(i)==uint32(0)      
        EmptyDataConfirm=true;
        break;     
    end
    
    
end

== matlab function PubIfDecisionTOS_MDL/TOS_20201112/TOS_2012080320/TOS/P0_Trajectory_V1.0/polyfit2 ==
  data: dx input; dy input; P0_Counter input; P0_EndPosition_dx input; P0_EndPosition_dy input; P0_TrgValidConfirm_Counter input; VxvRef_ms input; OTL_Valid output size=1; OTL_C3 output size=1; OTL_C2 output; OTL_C1 output size=1; OTL_C0 output size=1; OTL_Range output size=1; OTL_Cnt output size=1; d_Start output; d_End output; P0_Counter output size=80; dy output size=80; dx output size=80
function [ OTL_Valid,OTL_C3,OTL_C2,OTL_C1,OTL_C0,OTL_Range,OTL_Cnt,d_Start,d_End,P0_Counter,dy,dx] = ...
          fcn(dx,dy,P0_Counter, P0_EndPosition_dx, P0_EndPosition_dy, P0_TrgValidConfirm_Counter, VxvRef_ms)

%%-----初始化-----     


P0_Trajectory_TrackRecord_Num = uint32(80);

%%-----判断拟合点-----


%-----无效目标位补齐------
for i= uint32(1) : P0_Trajectory_TrackRecord_Num
    
        if dx(i)==single(0) && dy(i)==single(0) && P0_Counter(i)==uint32(0) 
            dx(i)=P0_EndPosition_dx;
            dy(i)=P0_EndPosition_dy;
        end
   
end


%----------判断起始、终止位置----------------------
% [min_dx,index_dx_min] = min(dx);
[min_dx,~] = min(dx);
[max_dy,~] = max(dx);
 d_End = max_dy;
 d_Start = min_dx;

% d_End = P0_EndPosition_dx;
% d_Start = P0_StartPosition_Dis;

%-----P0存在生命周期----
OTL_Cnt=uint8(P0_TrgValidConfirm_Counter);


%-------dop range--------
OTL_Range = single(max_dy) ;


%----------轨迹拟合----------------------
if d_Start< single(50) &&  VxvRef_ms >= 0.4166  && P0_TrgValidConfirm_Counter > uint8(5)
    P0_Trajectory_Line = polyfit(dx,dy,3);
    OTL_C3 = P0_Trajectory_Line(1);
    OTL_C2 = P0_Trajectory_Line(2);
    OTL_C1 = P0_Trajectory_Line(3);
    OTL_C0 = P0_Trajectory_Line(4); 
    OTL_Valid = true;
else
    OTL_C3=single(0);
    OTL_C2=single(0);
    OTL_C1=single(0);
    OTL_C0=single(0); 
    OTL_Valid = false;
end
